simulink model "PS4"  (R2018b)
settings: Solver=ode1  StartTime=0.0  StopTime=20  FixedStep=.001  RelTol=1e-3
values from neighbouring files (symbols this model uses):
  A = [0 0 0 -10 1 0 0 -1 0 1 0 -2 ... (16 elements, 4x4)]    [final2 FUNCIONA.mat]    (also in funcionaobservador.mat)
  A3 = [0  1  0; 0  0  1; 4374  -81  -36]    [final2 FUNCIONA.mat]    (also in funcionaobservador.mat)
  A9 = [0  1  0; 0  0  1; 1683  -439  37]    [final2 FUNCIONA.mat]    (also in funcionaobservador.mat)
  B = [0 0 0 1]    [final2 FUNCIONA.mat]    (also in funcionaobservador.mat)
  B3 = [0 0 1]    [final2 FUNCIONA.mat]    (also in funcionaobservador.mat)
  B9 = [0 0 1]    [final2 FUNCIONA.mat]    (also in funcionaobservador.mat)
  C = [13 7 0 0]    [final2 FUNCIONA.mat]    (also in funcionaobservador.mat)
  C3 = [39.6 4 0]    [final2 FUNCIONA.mat]    (also in funcionaobservador.mat)
  C3B = [1 0 0]    [final2 FUNCIONA.mat]    (also in funcionaobservador.mat)
  C9 = [10 0 0]    [final2 FUNCIONA.mat]    (also in funcionaobservador.mat)
  K = [110 153 69 11]    [final2 FUNCIONA.mat]    (also in funcionaobservador.mat)
  K3 = [4380 -70 -30]    [final2 FUNCIONA.mat]    (also in funcionaobservador.mat)
  K3B = [4380 -70 -30]    [final2 FUNCIONA.mat]    (also in funcionaobservador.mat)
  K9 = [1689 -428 43]    [final2 FUNCIONA.mat]    (also in funcionaobservador.mat)
  L3 = [0.25002206018 -3.22521839578 129.179662118]    [final2 FUNCIONA.mat]    (also in funcionaobservador.mat)
  L9 = [7 251.3 6525.4]    [final2 FUNCIONA.mat]    (also in funcionaobservador.mat)
libraries: cstblocks x2
settings Model: Creator=Abraham Pérez  LastModifiedBy=Abraham Pérez
settings SolverCC: InitialStep=.001

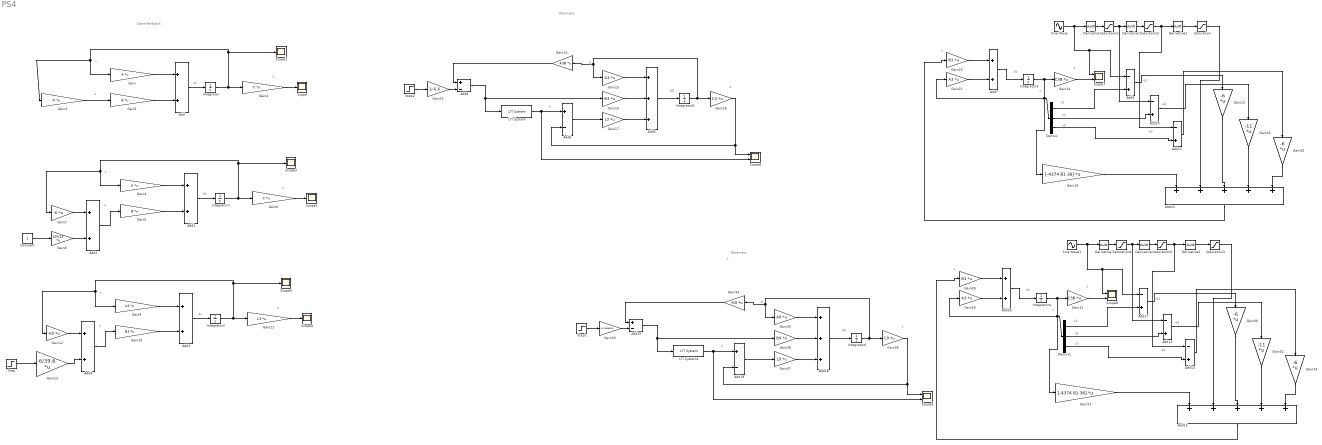
== system PS4 ==
  note: e3
  note: e2
  note: e1
  note: x3
  note: x2
  note: x1
  note: x
  note: u
  note: State feedback
  note: y
  note: dx
  note: u
  note: x
  note: dx
  note: y
  note: x
  note: u
  note: dx
  note: x
  note: y
  note: u
  note: Observers
  note: dO
  note: y
  note: s
  note: y
  note: O
  note: s
  note: dx
  note: e3
  note: u
  note: e1
  note: x2
  note: x1
  note: x
  note: s
  note: e2
  note: x3
  note: dx
  note: Observers
  note: y
  note: O
  note: s
  note: dO
  Add{,1..4,7,16} (7 alike) : Sum
  Add{9..11,13..14,17} (6 alike) : Sum  Inputs=-+
  Add12 : Sum  Inputs=+++++
  Add15 : Sum  Inputs=+++++
  Add18 : Sum  Inputs=+++
  Add{6,8,19..20} (4 alike) : Sum  Inputs=+-
  Add5 : Sum  Inputs=+++
  Constant : Constant
  Demux : Demux  Outputs=3
  Demux1 : Demux  Outputs=3
  Derivative{,1..5} (6 alike) : Derivative
  Gain : Gain  Gain=A  Multiplication=Matrix(K*u)
  Gain1 : Gain  Gain=B  Multiplication=Matrix(K*u)
  Gain{10,16,20,28} (4 alike) : Gain  Gain=B3  Multiplication=Matrix(K*u)
  Gain11 : Gain  Gain=C3  Multiplication=Matrix(K*u)
  Gain12 : Gain  Gain=-K3  Multiplication=Matrix(K*u)
  Gain13 : Gain  Gain=6/39.6  Multiplication=Matrix(K*u)
  Gain14 : Gain  Gain=-K3B  Multiplication=Matrix(K*u)
  Gain{9,15,21,29} (4 alike) : Gain  Gain=A3  Multiplication=Matrix(K*u)
  Gain17 : Gain  Gain=L3  Multiplication=Matrix(K*u)
  Gain18 : Gain  Gain=C3  Multiplication=Matrix(K*u)
  Gain19 : Gain  Gain=[-4374 81 36]  Multiplication=Matrix(K*u)
  Gain2 : Gain  Gain=C  Multiplication=Matrix(K*u)
  Gain22 : Gain  Gain=1/-6.6
  Gain{23,26,30,33} (4 alike) : Gain  Gain=-6  Multiplication=Matrix(K*u)
  Gain24 : Gain  Gain=C3B  Multiplication=Matrix(K*u)
  Gain25 : Gain  Gain=-11  Multiplication=Matrix(K*u)
  Gain27 : Gain  Gain=[-4374 81 36]  Multiplication=Matrix(K*u)
  Gain3 : Gain  Gain=-K  Multiplication=Matrix(K*u)
  Gain31 : Gain  Gain=C3B  Multiplication=Matrix(K*u)
  Gain32 : Gain  Gain=-11  Multiplication=Matrix(K*u)
  Gain34 : Gain  Gain=-K9  Multiplication=Matrix(K*u)
  Gain35 : Gain  Gain=A9  Multiplication=Matrix(K*u)
  Gain36 : Gain  Gain=B9  Multiplication=Matrix(K*u)
  Gain37 : Gain  Gain=L9  Multiplication=Matrix(K*u)
  Gain38 : Gain  Gain=C9  Multiplication=Matrix(K*u)
  Gain39 : Gain  Gain=1/-1.668429
  Gain4 : Gain  Gain=A  Multiplication=Matrix(K*u)
  Gain5 : Gain  Gain=B  Multiplication=Matrix(K*u)
  Gain6 : Gain  Gain=C  Multiplication=Matrix(K*u)
  Gain7 : Gain  Gain=-K  Multiplication=Matrix(K*u)
  Gain8 : Gain  Gain=120/13  Multiplication=Matrix(K*u)
  Integrator : Integrator  InitialCondition=[-1 .5 .5 1]
  Integrator1 : Integrator  InitialCondition=[-1 .5 .5 1]
  Integrator2 : Integrator  InitialCondition=[-1 .5 .5 ]
  Integrator{3..6} (4 alike) : Integrator  InitialCondition=[1 0 -1]
  LTI System : cstblocks/LTI System  sys=G3  IC=[]
  LTI System1 : cstblocks/LTI System  sys=G9  IC=[]
  Saturation{,1..5} (6 alike) : Saturate  UpperLimit=1  LowerLimit=-1
  Scope{,1..5} (6 alike) : Scope
  Scope{6..9} (4 alike) : Scope  NumInputPorts=2
  Sine Wave : Sin  Amplitude=.05  SampleTime=0
  Sine Wave1 : Sin  SampleTime=0
  Step : Step  After=26  SampleTime=0
  Step1 : Step  After=10  SampleTime=0
  Step2 : Step  After=52  SampleTime=0
  wires:
  Integrator/1 -> Gain2/1, Scope1/1, Gain/1, Gain3/1
  Gain/1 -> Add/1
  Gain1/1 -> Add/2
  Add/1 -> Integrator/1
  Gain2/1 -> Scope/1
  Gain3/1 -> Gain1/1
  Add1/1 -> Integrator1/1
  Integrator1/1 -> Gain6/1, Scope3/1, Gain4/1, Gain7/1
  Gain5/1 -> Add1/2
  Gain6/1 -> Scope2/1
  Gain4/1 -> Add1/1
  Gain7/1 -> Add2/1
  Add2/1 -> Gain5/1
  Gain8/1 -> Add2/2
  Constant/1 -> Gain8/1
  Step/1 -> Gain13/1
  Gain12/1 -> Add4/1
  Gain13/1 -> Add4/2
  Add4/1 -> Gain10/1
  Gain10/1 -> Add3/2
  Gain11/1 -> Scope4/1
  Gain9/1 -> Add3/1
  Add3/1 -> Integrator2/1
  Integrator2/1 -> Gain11/1, Scope5/1, Gain9/1, Gain12/1
  Gain17/1 -> Add5/3
  LTI System/1 -> Scope6/2, Add6/1
  Add6/1 -> Gain17/1
  Integrator5/1 -> Gain18/1, Gain15/1, Gain14/1
  Add5/1 -> Integrator5/1
  Gain15/1 -> Add5/1
  Gain16/1 -> Add5/2
  Gain14/1 -> Add8/1
  Gain22/1 -> Add8/2
  Step2/1 -> Gain22/1
  Add8/1 -> Gain16/1, LTI System/1
  Gain18/1 -> Scope6/1, Add6/2
  Gain20/1 -> Add7/1
  Add7/1 -> Integrator3/1
  Gain21/1 -> Add7/2
  Derivative1/1 -> Saturation2/1
  Demux/1 -> Add9/2
  Demux/2 -> Add10/2
  Demux/3 -> Add11/2
  Integrator3/1 -> Gain19/1, Gain21/1, Demux/1, Gain24/1
  Gain19/1 -> Add12/1
  Add9/1 -> Gain23/1
  Gain23/1 -> Add12/3
  Add10/1 -> Gain25/1
  Gain25/1 -> Add12/4
  Add11/1 -> Gain26/1
  Gain26/1 -> Add12/5
  Add12/1 -> Gain20/1
  Derivative2/1 -> Saturation/1
  Saturation2/1 -> Add11/1, Derivative2/1
  Saturation/1 -> Add12/2
  Gain24/1 -> Scope7/2
  Saturation1/1 -> Add10/1, Derivative1/1
  Derivative/1 -> Saturation1/1
  Sine Wave/1 -> Scope7/1, Add9/1, Derivative/1
  Add15/1 -> Gain28/1
  Gain30/1 -> Add15/3
  Gain28/1 -> Add16/1
  Add13/1 -> Gain32/1
  Derivative5/1 -> Saturation3/1
  Add14/1 -> Gain33/1
  Gain32/1 -> Add15/4
  Gain29/1 -> Add16/2
  Derivative4/1 -> Saturation5/1
  Integrator4/1 -> Gain27/1, Gain29/1, Demux1/1, Gain31/1
  Demux1/2 -> Add13/2
  Gain27/1 -> Add15/1
  Gain33/1 -> Add15/5
  Demux1/1 -> Add17/2
  Saturation5/1 -> Add14/1, Derivative5/1
  Gain31/1 -> Scope8/2
  Demux1/3 -> Add14/2
  Saturation4/1 -> Add13/1, Derivative4/1
  Derivative3/1 -> Saturation4/1
  Sine Wave1/1 -> Scope8/1, Add17/1, Derivative3/1
  Add17/1 -> Gain30/1
  Saturation3/1 -> Add15/2
  Add16/1 -> Integrator4/1
  Gain39/1 -> Add20/2
  LTI System1/1 -> Scope9/2, Add19/1
  Add18/1 -> Integrator6/1
  Integrator6/1 -> Gain38/1, Gain35/1, Gain34/1
  Gain37/1 -> Add18/3
  Gain36/1 -> Add18/2
  Step1/1 -> Gain39/1
  Gain34/1 -> Add20/1
  Add20/1 -> Gain36/1, LTI System1/1
  Gain35/1 -> Add18/1
  Gain38/1 -> Scope9/1, Add19/2
  Add19/1 -> Gain37/1
